simulink model "ITMBS_1m_M1"  (R2023a)
settings: Solver=FixedStepDiscrete  StartTime=0.0  StopTime=10.0  FixedStep=0.05  RelTol=1e-3  EnableMultiTasking=on
libraries: legoev3lib x4
settings Model: ExtModeTrigDuration=2  Creator=nikhil  LastModifiedBy=Sachin K S
settings SolverCC: PositivePriorityOrder=on  AutoInsertRateTranBlk=on
settings OptimizationCC: EnhancedBackFolding=on  PassReuseOutputArgsAs=Individual arguments  ZeroExternalMemoryAtStartup=off  ZeroInternalMemoryAtStartup=off  MaxStackSize=64  OptimizeBlockOrder=speed  DifferentSizesBufferReuse=on  OptimizationCustomize=off  EfficientTunableParamExpr=on
settings DebuggingCC: ParameterTunabilityLossMsg=error
settings HardwareCC: ProdBitPerPointer=32  ProdBitPerSizeT=32  ProdBitPerPtrDiffT=32  ProdLargestAtomicInteger=Long  ProdWordSize=32  ProdHWDeviceType=ARM Compatible->ARM 9  UseEmbeddedCoderFeatures=off  UseSimulinkCoderFeatures=off
settings SFSimCC: MATLABDynamicMemAlloc=off
settings RTWCC: Description=Embedded Coder  SystemTargetFile=ert.tlc  HardwareBoard=LEGO MINDSTORMS EV3  TLCOptions="-aInlineSetEventsForThisBaseRateFcn=TLC_FALSE -aSuppressMultiTaskScheduler=TLC_FALSE  -aRateBasedStepFcn=0"  TemplateMakefile=ert_default_tmf  Toolchain=Sourcery G++ Lite v2009q3
settings CodeAppCC: ForceParamTrailComments=on  IgnoreCustomStorageClasses=off  OperatorAnnotations=on  SimulinkDataObjDesc=on  SFDataObjDesc=on  InsertBlockDesc=on
settings ERTTargetCC: SupportContinuousTime=on  SupportNonInlinedSFcns=on  SupportVariableSizeSignals=on  ExtModeTransport=2  ExtModeStaticAlloc=on  ExtModeMexFile=ext_xcp  ExtModeIntrfLevel=Level2 - Open

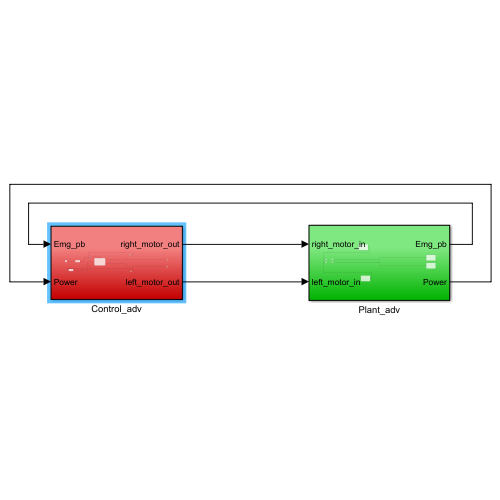
[thumbnail: Simulink's stored preview of the top-level diagram]
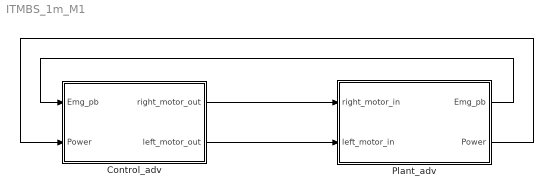
== system ITMBS_1m_M1 ==
  Control_adv : Subsystem
  Plant_adv : Subsystem
  wires:
  Control_adv/1(right_motor_out) -> Plant_adv/1(right_motor_in)
  Control_adv/2(left_motor_out) -> Plant_adv/2(left_motor_in)
  Plant_adv/1(Emg_pb) -> Control_adv/1(Emg_pb)
  Plant_adv/2(Power) -> Control_adv/2(Power)

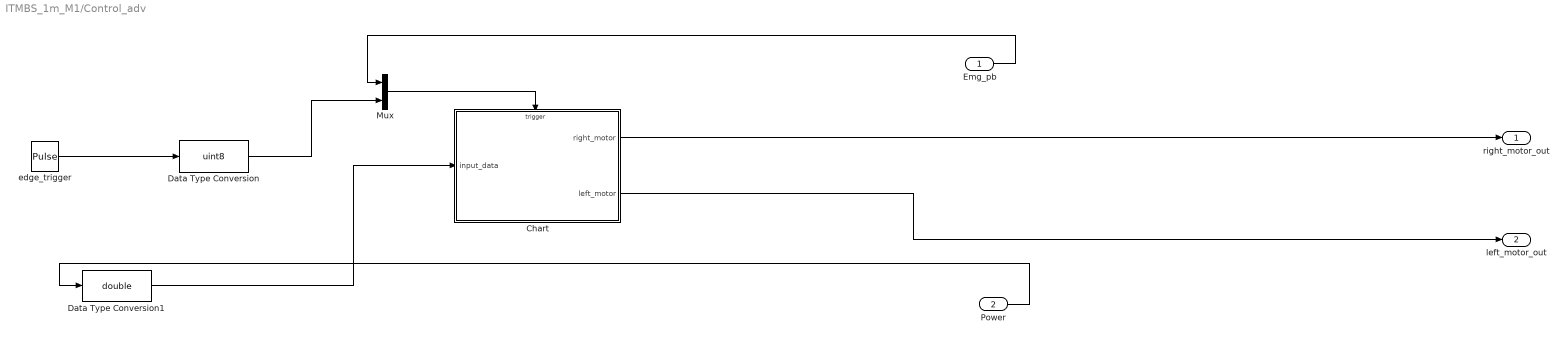
== system ITMBS_1m_M1/Control_adv ==
  Emg_pb : Inport
  Power : Inport  Port=2
  Chart : Stateflow chart  TreatAsAtomicUnit=on
  Data Type Conversion : DataTypeConversion  OutDataTypeStr=uint8  SaturateOnIntegerOverflow=off  RndMeth=Floor
  Data Type Conversion1 : DataTypeConversion  OutDataTypeStr=double  SaturateOnIntegerOverflow=off  RndMeth=Floor
  Mux : Mux  Inputs=2
  edge_trigger : DiscretePulseGenerator  Period=3  PulseWidth=2  SampleTime=0.05
  right_motor_out : Outport
  left_motor_out : Outport  Port=2
  wires:
  Emg_pb/1 -> Mux/1
  Data Type Conversion/1 -> Mux/2
  edge_trigger/1 -> Data Type Conversion/1
  Data Type Conversion1/1 -> Chart/1(input_data)
  Chart/2(left_motor) -> left_motor_out/1
  Chart/1(right_motor) -> right_motor_out/1
  Power/1 -> Data Type Conversion1/1
  Mux/1 -> Chart/Trigger

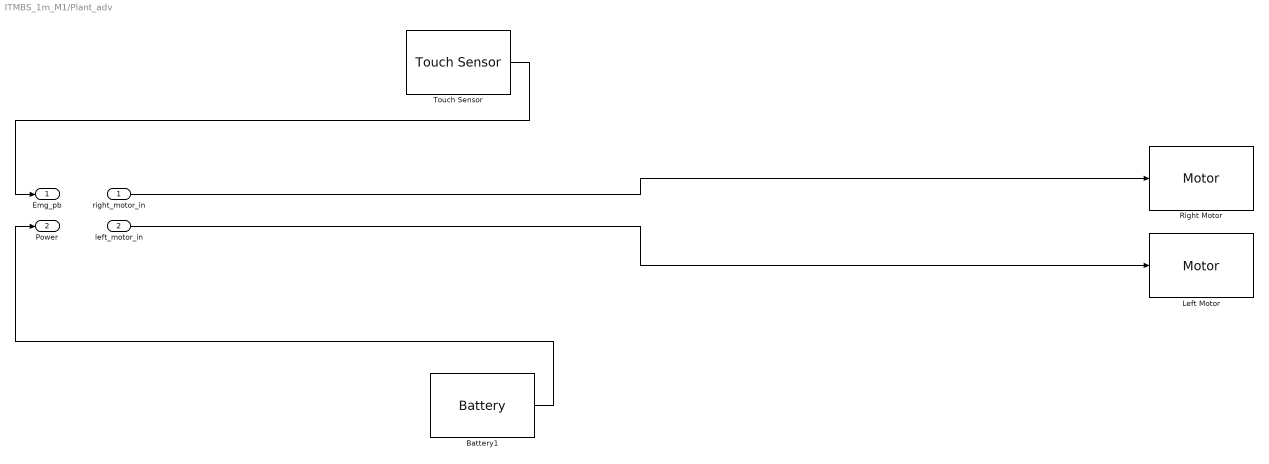
== system ITMBS_1m_M1/Plant_adv ==
  right_motor_in : Inport
  left_motor_in : Inport  Port=2
  Battery1 : legoev3lib/Battery  SampleTime=0.1
  Left Motor : legoev3lib/Motor  sportNumber=A  sstopAction=Brake
  Right Motor : legoev3lib/Motor  sportNumber=A  sstopAction=Brake
  Touch Sensor : legoev3lib/Touch Sensor  portNumber=1  sampleTime=0.1
  Emg_pb : Outport
  Power : Outport  Port=2
  wires:
  left_motor_in/1 -> Left Motor/1
  Battery1/1 -> Power/1
  right_motor_in/1 -> Right Motor/1
  Touch Sensor/1 -> Emg_pb/1

== stateflow chart ITMBS_1m_M1/Control_adv/Chart ==
  settings: executeAtInitialization=1
  state ON_1m
    right_motor=input_data;
    left_motor = input_data;
  state OFF_1m
    right_motor=0;
    left_motor=0;
    entry:
    c=0;
  (default) -> ON_1m
  ON_1m -> OFF_1m : pushbutton_event_input || (after(1.95,sec))
  (junction 38) -> ON_1m [order 1] : [c==2]
  OFF_1m -> (junction 36)
  (junction 36) -> (junction 37) [order 1] : [pushbutton_event_input]
  (junction 36) -> (junction 38) [order 2]
  (junction 37) -> (junction 39) : {c= c+1;}
  (junction 39) -> (junction 38)
  (junction 38) -> (junction 53) [order 2]
  data: input_data input; right_motor output; c local; left_motor output
  events: pushbutton_event_input input RISING_EDGE_EVENT; trigger input RISING_EDGE_EVENT
